simulink model "osservatore_4"  (R2019b)
settings: Solver=VariableStepAuto  StartTime=0.0  StopTime=20  MaxStep=1e-3  RelTol=1e-3
undefined symbols (not defined in the file): Ao, Bo, Co, L, Ts
libraries: cstblocks x1
settings Model: Creator=jacobi  LastModifiedBy=manue

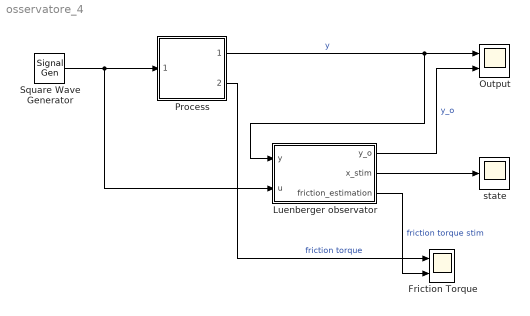
== system osservatore_4 ==
  Friction Torque : Scope  NumInputPorts=2
  Luenberger observator : Subsystem
  Output : Scope  NumInputPorts=2
  Process : Subsystem
  Square Wave Generator : SignalGenerator  WaveForm=square  Amplitude=4  Frequency=0.5  Units=rad/sec
  state : Scope
  wires:
  Luenberger observator/1(y_o) -> Output/2  "y_o"
  Luenberger observator/2(x_stim) -> state/1
  Square Wave Generator/1 -> Process/1(Torque), Luenberger observator/2(u)
  Process/1(Position) -> Luenberger observator/1(y), Output/1  "y"
  Process/2(Friction torque) -> Friction Torque/1  "friction torque"
  Luenberger observator/3(friction_estimation) -> Friction Torque/2  "friction torque stim"

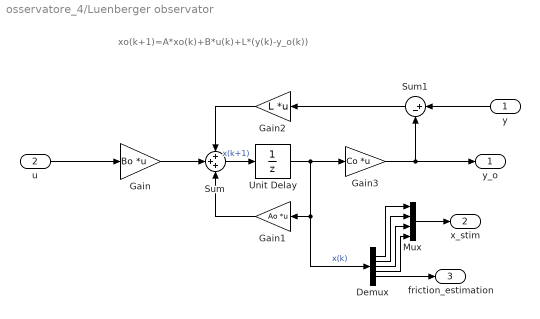
== system osservatore_4/Luenberger observator ==
  note: xo(k+1)=A*xo(k)+B*u(k)+L*(y(k)-y_o(k))
  y : Inport
  u : Inport  Port=2
  Demux : Demux  Outputs=5
  Gain : Gain  Gain=Bo  Multiplication=Matrix(K*u)
  Gain1 : Gain  Gain=Ao  Multiplication=Matrix(K*u)
  Gain2 : Gain  Gain=L  Multiplication=Matrix(K*u)
  Gain3 : Gain  Gain=Co  Multiplication=Matrix(K*u)
  Mux : Mux
  Sum : Sum  Inputs=+++
  Sum1 : Sum  Inputs=|+-
  Unit Delay : UnitDelay  SampleTime=Ts  HasFrameUpgradeWarning=on
  y_o : Outport
  x_stim : Outport  Port=2
  friction_estimation : Outport  Port=3
  wires:
  Unit Delay/1 -> Gain3/1, Demux/1, Gain1/1  "x(k)"
  Sum/1 -> Unit Delay/1  "x(k+1)"
  Gain1/1 -> Sum/3
  Gain/1 -> Sum/2
  Gain3/1 -> Sum1/2, y_o/1
  Sum1/1 -> Gain2/1
  Gain2/1 -> Sum/1
  u/1 -> Gain/1
  y/1 -> Sum1/1
  Demux/5 -> friction_estimation/1
  Demux/4 -> Mux/4
  Demux/3 -> Mux/3
  Demux/2 -> Mux/2
  Demux/1 -> Mux/1
  Mux/1 -> x_stim/1

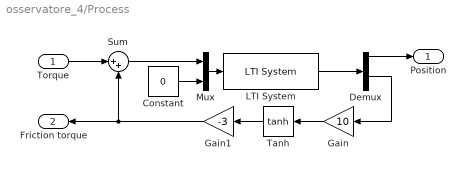
== system osservatore_4/Process ==
  Torque : Inport
  Constant : Constant  Value=0
  Demux : Demux
  Gain : Gain  Gain=10
  Gain1 : Gain  Gain=-3
  LTI System : cstblocks/LTI System  sys=model  IC=[]
  Mux : Mux  Inputs=2
  Sum : Sum  Inputs=|++
  Tanh : Trigonometry  Operator=tanh
  Position : Outport
  Friction torque : Outport  Port=2
  wires:
  Sum/1 -> Mux/1
  Torque/1 -> Sum/1
  LTI System/1 -> Demux/1
  Demux/1 -> Position/1
  Demux/3 -> Gain/1
  Tanh/1 -> Gain1/1
  Gain/1 -> Tanh/1
  Gain1/1 -> Friction torque/1, Sum/2
  Mux/1 -> LTI System/1
  Constant/1 -> Mux/2
